simulink model "ML_UAV_3D_2"  (R2018a)
settings: Solver=ode4  StartTime=0.0  StopTime=130  FixedStep=Ts  MaxStep=2*T  MinStep=T  RelTol=1e-4
values from neighbouring files (symbols this model uses):
  Ac = 0.0331    [init_ML_UAV_3D_2.m]
  Am1_LPF = sysd.denominator{1}    [init_ML_UAV_3D_2.m]
  Am2_LPF = sysd.denominator{1}    [init_ML_UAV_3D_2.m]
  Am_coup_LPF = sysd.denominator{1}    [init_ML_UAV_3D_2.m]
  Amp_sf = 3    [init_ML_UAV_3D_2.m]
  Amp_sf_rp = 0.05*uav.m*g    [init_ML_UAV_3D_2.m]
  Bm1_LPF = sysd.numerator{1}    [init_ML_UAV_3D_2.m]
  Bm2_LPF = sysd.numerator{1}    [init_ML_UAV_3D_2.m]
  Bm_coup_LPF = sysd.numerator{1}    [init_ML_UAV_3D_2.m]
  C_S = [5;5;9]*10^-3    [init_ML_UAV_3D_2.m]
  Cd_u = 0.2    [init_ML_UAV_3D_2.m]
  dc_M_p = 6.7    [init_ML_UAV_3D_2.m]
  eps_V = 0.5    [init_ML_UAV_3D_2.m]
  g = 9.81    [init_ML_UAV_3D_2.m]
  gamma_d_p = (2*0.3/0.03*2*0.2*12/4)/10    (= 2.4)    [init_ML_UAV_3D_2.m]
  k3 = 24    [init_ML_UAV_3D_2.m]
  k4 = 0.8    [init_ML_UAV_3D_2.m]
  min_sf = 5    [init_ML_UAV_3D_2.m]
  min_sf_rp = 0.35*uav.m*g    [init_ML_UAV_3D_2.m]
  OMEGA_FILTER_OUTER = 40    [estimation.m]
  T_init = 10    [init_ML_UAV_3D_2.m]
  Tc = 1/500    (= 0.002)    [estimation.m]
  Tg = 1/ 20    (= 0.05)    [estimation.m]
  Tn = 1/500    (= 0.002)    [estimation.m]
  Ts = 1/500    (= 0.002)    [estimation.m]    (also in init_ML_UAV_3D_2.m)
  Tsc = 1/100    (= 0.01)    [estimation.m]
  Tz = 1/500    (= 0.002)    [estimation.m]
  X_GPS_offset = [0.01 0.005]    [estimation.m]
undefined symbols (not defined in the file or in its folder): Am_HPF, Am_LPF, Am_LPF2, an1, an1_v, an2, an3, Bm_HPF, Bm_LPF, Bm_LPF2, bn1, bn1_v, bn2, bn3, buoy, cable, controller, current, D_b, DiscIntNeverNeededParam, F, filters, J_u, K, kd_t, kp_t, L, Light, magnitude, MIL, Phi0, Psi0, R_b, T, Theta0, theta_q_ini, tolerences, torque_corr, uav, Vol_b, water, wave, X0_u
libraries: simulink x48, simulink_extras x10, UAV_Control x4, dspmtrx3 x2, aerolibwind2 x2
(part 4 of 6)

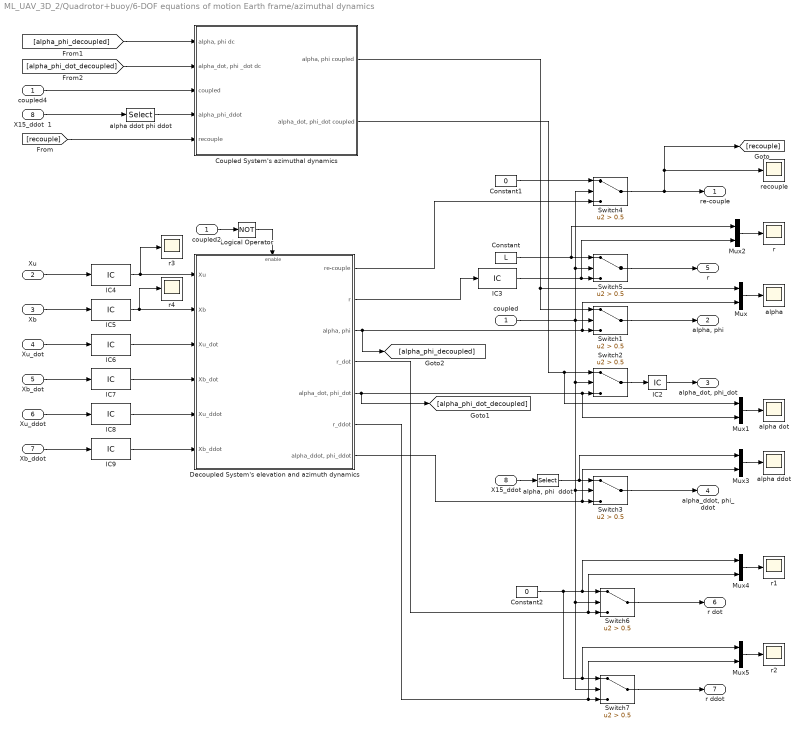
== system ML_UAV_3D_2/Quadrotor+buoy/6-DOF equations of motion Earth frame/azimuthal dynamics ==
  coupled : Inport
  Xu : Inport  Port=2
  Xb : Inport  Port=3
  "Xu_dot " : Inport  Port=4
  Xb_dot : Inport  Port=5
  Xu_ddot : Inport  Port=6
  "Xb_ddot   " : Inport  Port=7
  "X15_ddot  " : Inport  Port=8
  "    alpha ddot" : Scope
  "  alpha" : Scope
  "  alpha dot" : Scope
    r{,1..4} (5 alike) : Scope
  "  recouple   " : Scope
  Constant : Constant  Value=L
  Constant1 : Constant  Value=0
  Constant2 : Constant  Value=0
  Coupled System's azimuthal dynamics : Subsystem
  Decoupled System's elevation and azimuth dynamics : Subsystem  TreatAsAtomicUnit=on
  IC2 : InitialCondition  Value=0
  IC3 : InitialCondition  Value=r_0
  IC4 : InitialCondition  Value=pos_u_ini
  IC5 : InitialCondition  Value=pos_b_ini
  IC6 : InitialCondition  Value=v_u_ini
  IC7 : InitialCondition  Value=v_b_ini
  IC8 : InitialCondition  Value=[0; 0; 0]
  IC9 : InitialCondition  Value=[0; 0; 0]
  Logical Operator : Logic  Operator=NOT  AllPortsSameDT=off  OutDataTypeStr=boolean
  Mux{,1..5} (6 alike) : Mux  Inputs=2
  Switch{1..7} (7 alike) : Switch  Criteria=u2 > Threshold  Threshold=0.5
  X15_ddot  1 : InportShadow  Port=8
  alpha ddot phi ddot : Selector  InputPortWidth=5  IndexOptions=Index vector (dialog)  Indices=[4 5]  OutputSizes=1
  "alpha, phi  ddot" : Selector  InputPortWidth=5  IndexOptions=Index vector (dialog)  Indices=[4 5]  OutputSizes=1
  coupled2 : InportShadow
  coupled4 : InportShadow
  re-couple : Outport
  "alpha, phi" : Outport  Port=2
  "alpha_dot, phi_dot " : Outport  Port=3
  "alpha_ddot, phi_ddot" : Outport  Port=4
  "r " : Outport  Port=5
  r dot : Outport  Port=6
  r ddot : Outport  Port=7
  wires:
  coupled/1 -> Switch7/2, Switch6/2, Switch3/2, Switch2/2, Switch4/2, Switch5/2, Switch1/2
  "X15_ddot  "/1 -> "alpha, phi  ddot"/1
  Switch3/1 -> "alpha_ddot, phi_ddot"/1
  Coupled System's azimuthal dynamics/2("alpha_dot, phi_dot coupled") -> Switch2/1, Mux1/1
  Switch2/1 -> IC2/1
  Xb/1 -> IC5/1
  Xu/1 -> IC4/1
  alpha ddot phi ddot/1 -> Coupled System's azimuthal dynamics/4(alpha_phi_ddot)
  [alpha_phi_dot_decoupled] -> Coupled System's azimuthal dynamics/2("alpha_dot, phi _dot dc")
  coupled4/1 -> Coupled System's azimuthal dynamics/3(coupled)
  [alpha_phi_decoupled] -> Coupled System's azimuthal dynamics/1("alpha, phi dc")
  X15_ddot  1/1 -> alpha ddot phi ddot/1
  "Xu_dot "/1 -> IC6/1
  Xb_dot/1 -> IC7/1
  "Xb_ddot   "/1 -> IC9/1
  Xu_ddot/1 -> IC8/1
  coupled2/1 -> Logical Operator/1
  Switch5/1 -> "r "/1
  Constant/1 -> Switch5/1, Mux2/1
  Decoupled System's elevation and azimuth dynamics/2(r) -> IC3/1
  [recouple] -> Coupled System's azimuthal dynamics/5(recouple)
  Coupled System's azimuthal dynamics/1("alpha, phi coupled") -> Mux/1, Switch1/1
  Decoupled System's elevation and azimuth dynamics/7("alpha_ddot, phi_ddot") -> Mux3/2, Switch3/3
  Logical Operator/1 -> Decoupled System's elevation and azimuth dynamics/Enable
  Mux/1 -> "  alpha"/1
  Mux1/1 -> "  alpha dot"/1
  Decoupled System's elevation and azimuth dynamics/5("alpha_dot, phi_dot") -> Mux1/2, Switch2/3, [alpha_phi_dot_decoupled]
  Mux2/1 -> "  r"/1
  Decoupled System's elevation and azimuth dynamics/1(re-couple) -> Switch4/3
  Mux3/1 -> "    alpha ddot"/1
  "alpha, phi  ddot"/1 -> Mux3/1, Switch3/1
  Switch4/1 -> [recouple], "  recouple   "/1, re-couple/1
  Constant1/1 -> Switch4/1
  Switch1/1 -> "alpha, phi"/1
  IC2/1 -> "alpha_dot, phi_dot "/1
  Mux4/1 -> "  r1"/1
  Switch6/1 -> r dot/1
  Decoupled System's elevation and azimuth dynamics/4(r_dot) -> Mux4/2, Switch6/3
  Decoupled System's elevation and azimuth dynamics/6(r_ddot) -> Switch7/3, Mux5/2
  Constant2/1 -> Switch7/1, Mux5/1, Mux4/1, Switch6/1
  Switch7/1 -> r ddot/1
  Mux5/1 -> "  r2"/1
  IC3/1 -> Mux2/2, Switch5/3
  IC4/1 -> "  r3"/1, Decoupled System's elevation and azimuth dynamics/1(Xu)
  IC6/1 -> Decoupled System's elevation and azimuth dynamics/3(Xu_dot)
  IC7/1 -> Decoupled System's elevation and azimuth dynamics/4(Xb_dot)
  IC8/1 -> Decoupled System's elevation and azimuth dynamics/5(Xu_ddot)
  IC9/1 -> Decoupled System's elevation and azimuth dynamics/6(Xb_ddot)
  Decoupled System's elevation and azimuth dynamics/3("alpha, phi") -> Switch1/3, Mux/2, [alpha_phi_decoupled]
  IC5/1 -> "  r4"/1, Decoupled System's elevation and azimuth dynamics/2(Xb)

== system ML_UAV_3D_2/Quadrotor+buoy/6-DOF equations of motion Earth frame/buoyancy ==
  z_b : Inport
  zeta : Inport  Port=2
  Constant : Constant  Commented=on  Value=g*rho_w*l_b*R_b
  Manual Switch : ManualSwitch  CurrentSetting=0
  Product : Product  Commented=on
  Scope1 : Scope  Commented=on
  Scope3 : Scope  Commented=on
  V_im cuboid : Subsystem
  f(z_b,zeta) cylinder : Subsystem  Commented=on
  two connected cylindrical buoys : Gain  Commented=on  Gain=2
  two connected cylindrical buoys1 : Gain  Commented=on  Gain=l_b*R_b
  two connected cylindrical buoys2 : Gain  Commented=on  Gain=2
  V_im : Outport
  wires:
  z_b/1 -> V_im cuboid/2(zb), f(z_b,zeta) cylinder/2(zb)
  zeta/1 -> V_im cuboid/1(zeta), f(z_b,zeta) cylinder/1(zeta)
  Product/1 -> two connected cylindrical buoys/1
  Constant/1 -> Scope1/1, Product/2
  f(z_b,zeta) cylinder/1(Out1) -> two connected cylindrical buoys1/1, Product/1, Scope3/1
  Manual Switch/1 -> V_im/1
  V_im cuboid/1(Vol_im) -> Manual Switch/2
  two connected cylindrical buoys1/1 -> two connected cylindrical buoys2/1
  two connected cylindrical buoys2/1 -> Manual Switch/1

== system ML_UAV_3D_2/Quadrotor+buoy/6-DOF equations of motion Earth frame/elevation and azimuth angles to Direction Cosine Matrix Spherical to Cartesian ==
  "alpha, phi" : Inport
  -s_alpha*c_phi : Fcn  Expr=-u(1)*u(4)
  -s_alpha*s_phi : Fcn  Expr=-u(1)*u(2)
  -s_phi : Fcn  Expr=-u(2)
  Ground : Ground
  Mux : Mux  Inputs=2
  Subsystem : Subsystem
  c_alpha : Fcn  Expr=u(3)
  c_alpha*c_phi : Fcn  Expr=u(3)*u(4)
  c_alpha*s_phi : Fcn  Expr=u(3)*u(2)
  c_phi : Fcn  Expr=u(4)
  s_alpha : Fcn  Expr=u(1)
  sincos : Trigonometry  Operator=sincos
  DCM : Outport  PortDimensions=[3,3]
  wires:
  -s_alpha*c_phi/1 -> Subsystem/2(In2)
  -s_phi/1 -> Subsystem/3(In3)
  Subsystem/1(Out1) -> DCM/1
  c_alpha/1 -> Subsystem/8(In8)
  sincos/2 -> Mux/2
  s_alpha/1 -> Subsystem/7(In7)
  c_alpha*s_phi/1 -> Subsystem/4(In4)
  Ground/1 -> Subsystem/9(In9)
  Mux/1 -> c_alpha*s_phi/1, s_alpha/1, c_alpha/1, c_phi/1, -s_alpha*s_phi/1, -s_phi/1, -s_alpha*c_phi/1, c_alpha*c_phi/1
  -s_alpha*s_phi/1 -> Subsystem/5(In5)
  c_alpha*c_phi/1 -> Subsystem/1(In1)
  c_phi/1 -> Subsystem/6(In6)
  sincos/1 -> Mux/1
  "alpha, phi"/1 -> sincos/1

== system ML_UAV_3D_2/Quadrotor+buoy/6-DOF equations of motion Earth frame/u123 ==
  u1 : Inport
  euler_u : Inport  Port=2
  V_im : Inport  Port=3
  a_p : Inport  Port=4
  coupled : Inport  Port=5
  -s_alpha*c_phi : Fcn  Expr=-u(1)*u(4)
  -s_alpha*s_phi : Fcn  Expr=-u(1)*u(2)
  Add : Sum
  Add1 : Sum  Inputs=3
  Constant1 : Constant  Value=rho_w*g
  Constant2 : Constant  Commented=on  Value=Vol_b/2
  F_B : Product
  Gain : Gain  Gain=L
  Gain1 : Gain  Gain=L
  Mux : Mux  Inputs=2
  Mux1 : Mux  Inputs=2
  Mux2 : Mux  Inputs=3
  Product1 : Product  Inputs=3  SaturateOnIntegerOverflow=on  InputSameDT=on  OutDataTypeStr=Inherit: Same as first input
  Product{2..10} (9 alike) : Product  Inputs=**  SaturateOnIntegerOverflow=on  InputSameDT=on  OutDataTypeStr=Inherit: Same as first input
  Product11 : Product  Inputs=3  SaturateOnIntegerOverflow=on  InputSameDT=on  OutDataTypeStr=Inherit: Same as first input
  Scope{1..4,9} (5 alike) : Scope
  Signal Specification2 : SignalSpecification  Dimensions=5
  Sum1 : Sum  Inputs=|++  SaturateOnIntegerOverflow=on
  Vector Concatenate3 : Concatenate  NumInputs=5
  c_alpha : Fcn  Expr=u(3)
  c_phi : Fcn  Expr=u(4)
  c_phi c_theta : Fcn  Expr=u(4)*u(5)
  coupled1 : InportShadow  Port=5
  s_phi : Fcn  Expr=-u(2)
  s_theta c_psi + s_phi c_theta s_psi : Fcn  Expr=u(1)*u(5)*u(3) + u(2)*u(6)
  s_theta s_psi - s_phi c_theta c_psi : Fcn  Expr=-u(1)*u(5)*u(6) + u(2)*u(3)
  sincos : Trigonometry  Operator=sincos
  sincos1 : Trigonometry  Operator=sincos
  "u1 " : InportShadow
  u15 : Outport
  R_u_3 : Outport  Port=2
  wires:
  Product7/1 -> Sum1/1
  Product2/1 -> Product7/1, Product3/1, Product6/1
  Product1/1 -> Vector Concatenate3/4
  Vector Concatenate3/1 -> Scope9/1, Signal Specification2/1
  Product6/1 -> Vector Concatenate3/1
  Sum1/1 -> Vector Concatenate3/3
  F_B/1 -> Sum1/2
  V_im/1 -> F_B/1
  Gain/1 -> Product1/2
  Constant1/1 -> F_B/2
  Signal Specification2/1 -> u15/1
  coupled/1 -> Product2/1
  u1/1 -> Product2/2
  "u1 "/1 -> Product11/3, Product1/3
  Mux/1 -> c_phi c_theta/1, s_theta s_psi - s_phi c_theta c_psi/1, s_theta c_psi + s_phi c_theta s_psi/1
  sincos/1 -> Mux/1
  sincos/2 -> Mux/2
  euler_u/1 -> sincos/1
  s_theta c_psi + s_phi c_theta s_psi/1 -> Product9/1, Scope3/1, Product4/1, Mux2/1, Product6/2  "R_31"
  s_theta s_psi - s_phi c_theta c_psi/1 -> Scope4/1, Product10/1, Product5/1, Mux2/2, Product3/2  "R_32"
  Product3/1 -> Vector Concatenate3/2
  c_phi c_theta/1 -> Product8/1, Mux2/3, Product7/2  "R_33"
  a_p/1 -> sincos1/1
  sincos1/1 -> Mux1/1
  sincos1/2 -> Mux1/2
  Mux1/1 -> c_phi/1, s_phi/1, c_alpha/1, -s_alpha*s_phi/1, -s_alpha*c_phi/1
  -s_alpha*c_phi/1 -> Product4/2
  Product4/1 -> Add1/1
  Product5/1 -> Add1/2
  -s_alpha*s_phi/1 -> Product5/2
  Product8/1 -> Add1/3
  c_alpha/1 -> Product8/2
  Product9/1 -> Scope2/1, Add/1
  Product10/1 -> Scope1/1, Add/2
  s_phi/1 -> Product9/2
  c_phi/1 -> Product10/2
  Add1/1 -> Gain/1
  coupled1/1 -> Product11/1, Product1/1
  Gain1/1 -> Product11/2
  Product11/1 -> Vector Concatenate3/5
  Add/1 -> Gain1/1
  Mux2/1 -> R_u_3/1

== system ML_UAV_3D_2/Sensors and Filters/Coupling detection by r/Coupling state ==
  r_est : Inport
  re_couple : Inport  Port=2
  Data Type Conversion : DataTypeConversion  OutDataTypeStr=double
  Delay10 : Delay  DelayLength=1  InitialCondition=0
  IC3 : InitialCondition  Value=0
  IC5 : InitialCondition  Value=0
  MATLAB Function : MATLAB Function  TreatAsAtomicUnit=on
  "T, r,xu,xb1" : Scope
  break algebraic loop : Delay  DelayLength=1  InitialCondition=1
  cable length with safety margine1 : simulink/Logic and Bit Operations/Compare To Constant  relop=>=  const=cable.L_0-0.05  OutDataTypeStr=boolean
  "is coupled " : Scope
  is coupled -1 : Scope
  pos tension : Scope
  positive tension : Scope
  "re_couple " : Scope
  state detector : Scope
  is coupled : Outport
  wires:
  Delay10/1 -> is coupled -1/1, MATLAB Function/3(coupled)
  IC5/1 -> is coupled/1, Delay10/1
  MATLAB Function/1(is_coupled) -> IC5/1, "is coupled "/1
  break algebraic loop/1 -> pos tension/1, MATLAB Function/1(pos_T)
  re_couple/1 -> MATLAB Function/2(re_couple), "re_couple "/1
  MATLAB Function/2(c) -> state detector/1
  Data Type Conversion/1 -> positive tension/1, break algebraic loop/1
  IC3/1 -> Data Type Conversion/1
  cable length with safety margine1/1 -> IC3/1
  r_est/1 -> "T, r,xu,xb1"/1, cable length with safety margine1/1

== system ML_UAV_3D_2/Sensors and Filters/Data processing/Estimate Attitude ==
  Acc : Inport
  q : Inport  Port=2
  Euler : Inport  Port=3
  Calculate Roll and Pitch (From Acceleration Data) : Subsystem
  Constant : Constant  Value=Ts
  Demux : Demux  Outputs=2
  Ground : Ground
  High Pass Filter1 : DiscreteTransferFcn  Numerator=Bm_HPF  Denominator=Am_HPF
  Kalman Filter - Pitch : MATLAB Function  TreatAsAtomicUnit=on
  Manual Switch1 : ManualSwitch  CurrentSetting=0
  Mux : Mux  Inputs=3
  Mux2 : Mux  Inputs=2
  Mux5 : Mux  Inputs=2
  Notch Filter1 : Subsystem
  Scope1 : Scope
  Signal Specification : SignalSpecification  Dimensions=1
  theta : Scope
  q_g : Outport
  q_f : Outport  Port=2
  " pitch" : Outport  Port=3
  wires:
  q/1 -> High Pass Filter1/1, Mux2/2
  Notch Filter1/2(q) -> Kalman Filter - Pitch/2(gyro_rate), q_f/1
  Calculate Roll and Pitch (From Acceleration Data)/1(pitch_acc (rad)) -> Kalman Filter - Pitch/1(acc_angle)
  Signal Specification/1 -> " pitch"/1  "Kalman"
  Euler/1 -> Mux5/1, Kalman Filter - Pitch/3(opti_angle)  "pitch"
  Constant/1 -> Kalman Filter - Pitch/4(dt)
  Acc/1 -> Demux/1
  Notch Filter1/1(y) -> Manual Switch1/2
  High Pass Filter1/1 -> Manual Switch1/1, Notch Filter1/1(u), Mux2/1
  Mux2/1 -> Scope1/1
  Kalman Filter - Pitch/1(angle) -> Mux5/2, Signal Specification/1
  Mux/1 -> Calculate Roll and Pitch (From Acceleration Data)/1(accel (m/s^2) [3])
  Demux/1 -> Mux/1
  Demux/2 -> Mux/3
  Ground/1 -> Mux/2
  Manual Switch1/1 -> q_g/1
  Mux5/1 -> theta/1

== system ML_UAV_3D_2/Sensors and Filters/Data processing/Estimate Position ==
  OptiTrack : Inport
  "pitch, Kalman" : Inport  Port=2
  Sonar : Inport  Port=3
  2nd Order Filter : Subsystem
  2nd Order Filter2 : Subsystem
  2nd Order Filter4 : Subsystem
  2nd Order Filter5 : Subsystem
  Constant4 : Constant  Value=Tc
  Demux2 : Demux
  Extrapolation - x : MATLAB Function  TreatAsAtomicUnit=on
  Extrapolation - z : MATLAB Function  TreatAsAtomicUnit=on
  Height est : Scope
  Height est1 : Scope
  Kalman Filter - Height : MATLAB Function  TreatAsAtomicUnit=on
  Manual Switch : ManualSwitch  CurrentSetting=0
  Mux : Mux  Inputs=2
  Mux1 : Mux  Inputs=2
  Mux2 : Mux  Inputs=3
  Mux3 : Mux  Inputs=3
  Mux4 : Mux  Inputs=3
  Notch Filter2 : Subsystem
  Position : Selector  InputPortWidth=5  IndexOptions=Index vector (dialog)  Indices=[1 2 4 5]  OutputSizes=1
  Signal Conditioning - Sonar : Subsystem
  Signal Specification : SignalSpecification  Dimensions=2
  Signal Specification1 : SignalSpecification  Dimensions=2
  Step Size : Constant  Value=Tc
  Step Size1 : Constant  Value=X0_u(1)
  Step Size2 : Constant  Value=X0_u(2)
  Step Size3 : Constant  Value=X0_u(2)
  Terminator1 : Terminator
  Terminator2 : Terminator
  Thrust1 : Scope
  Thrust11 : Scope
  V_est : Scope  Commented=on
  X_est : Scope  Commented=on
  Xe : Outport
  Ve : Outport  Port=2
  wires:
  Demux2/1 -> Mux3/1, Extrapolation - x/1(xin)
  2nd Order Filter5/2(yd) -> [height_rate_Kalman]
  Demux2/3 -> Extrapolation - x/4(new), Extrapolation - z/4(new)  "New Data"
  Constant4/1 -> Kalman Filter - Height/3(dt)
  Extrapolation - x/1(xout) -> Mux3/2, 2nd Order Filter/1(u)
  2nd Order Filter/1(y) -> Mux3/3, Mux/1
  2nd Order Filter4/2(yd) -> Kalman Filter - Height/2(sonar_d)
  2nd Order Filter2/1(y) -> Mux4/3, Kalman Filter - Height/1(optitrack), Mux2/2
  Sonar/1 -> Signal Conditioning - Sonar/1(sonar (m))
  2nd Order Filter4/1(y) -> Terminator1/1
  Signal Conditioning - Sonar/1(calib sonar (m)) -> Mux2/1, 2nd Order Filter4/1(u)
  Step Size/1 -> Extrapolation - z/3(dt), Extrapolation - x/3(dt)
  Position/1 -> Demux2/1
  Demux2/2 -> Mux4/1, Extrapolation - z/1(xin)
  2nd Order Filter5/1(y) -> Terminator2/1
  Mux/1 -> Signal Specification/1  "Xe IMU or GPS"
  [height_rate_Kalman] -> Mux1/2
  Demux2/4 -> Extrapolation - x/5(isTracking), Extrapolation - z/5(isTracking)  "Is Tracking"
  Mux2/1 -> Height est/1
  Mux1/1 -> Signal Specification1/1  "Ve IMU or GPS"
  OptiTrack/1 -> Thrust1/1, Position/1
  Mux3/1 -> Thrust11/1
  2nd Order Filter2/2(yd) -> Extrapolation - z/2(xdotin)
  Notch Filter2/1(y) -> Manual Switch/2
  2nd Order Filter/2(yd) -> Notch Filter2/1(u), Manual Switch/1, Extrapolation - x/2(xdotin)
  Manual Switch/1 -> Mux1/1
  Signal Specification/1 -> Xe/1, X_est/1
  Signal Specification1/1 -> Ve/1, V_est/1
  Kalman Filter - Height/1(height) -> [height_Kalman], Mux2/3, 2nd Order Filter5/1(u)
  [height_Kalman] -> Mux/2
  "pitch, Kalman"/1 -> Signal Conditioning - Sonar/2(pitch (rad))
  Mux4/1 -> Height est1/1
  Extrapolation - z/1(xout) -> Mux4/2, 2nd Order Filter2/1(u)
  Step Size1/1 -> Extrapolation - x/6(x0)
  Step Size2/1 -> Extrapolation - z/6(x0)
  Step Size3/1 -> Kalman Filter - Height/4(x0)

== system ML_UAV_3D_2/Sensors and Filters/Sensors/ Sonar (10Hz) (true elevation instead real sonar signal) ==
  note: "Smooth" out the Sonar data
  note: Resample the 10Hz Sonar Data
  sonar (m) : Inport
  FOH1 : Subsystem  mask{Ts=0.1}
      mask prompts: Ts "Sample Time"
  IC : InitialCondition  Value=X0_u(2)
  Rate Transition : RateTransition  InitialCondition=X0_u(2)
  Sampler : Subsystem  mask{Ts=0.1}
      mask prompts: Ts "Sample Time"
  calib sonar (m) : Outport
  wires:
  Sampler/1(Out1) -> Rate Transition/1
  Rate Transition/1 -> FOH1/1(Input)
  sonar (m)/1 -> Sampler/1(In1)
  FOH1/1(Output) -> IC/1
  IC/1 -> calib sonar (m)/1

== system ML_UAV_3D_2/Sensors and Filters/Sensors/Accelerometer (500Hz) ==
  Ab : Inport
  "Ab " : Scope  Commented=on
  Demux1 : Demux  Outputs=2
  From File : FromFile  FileName=acc_x_noise.mat  SampleTime=Tz
  From File2 : FromFile  FileName=acc_z_noise.mat  SampleTime=Tz
  IC : InitialCondition  Value=[0 0]
  Manual Switch{,2,4,6} (4 alike) : ManualSwitch
  Mux1 : Mux  Inputs=2
  Mux2 : Mux  Inputs=2
  Product : Product  SaturateOnIntegerOverflow=on  RndMeth=Zero  InputSameDT=on  OutDataTypeStr=Inherit: Same as first input
  Product2 : Product  SaturateOnIntegerOverflow=on  RndMeth=Zero  InputSameDT=on  OutDataTypeStr=Inherit: Same as first input
  Slider Gain : simulink/Math Operations/Slider Gain  gain=1  low=0  high=2
  Slider Gain2 : simulink/Math Operations/Slider Gain  gain=1  low=0  high=2
  Sum2 : Sum  Inputs=+++  SaturateOnIntegerOverflow=on  InputSameDT=on  OutDataTypeStr=Inherit: Same as first input
  Sum5 : Sum  Inputs=+++  SaturateOnIntegerOverflow=on  InputSameDT=on  OutDataTypeStr=Inherit: Same as first input
  acc_noisy : Scope  Commented=on
  bias : Constant  Value=0.05  VectorParams1D=off
  bias10 : Constant  Value=1.02  VectorParams1D=off
  bias11 : Constant  VectorParams1D=off
  bias3 : Constant  Value=1.02  VectorParams1D=off
  bias4 : Constant  VectorParams1D=off
  bias6 : Constant  Value=0  VectorParams1D=off
  bias7 : Constant  Value=0.05  VectorParams1D=off
  bias8 : Constant  Value=0  VectorParams1D=off
  Acc : Outport
  wires:
  bias11/1 -> Manual Switch6/2
  bias10/1 -> Manual Switch6/1
  bias4/1 -> Manual Switch4/2
  bias3/1 -> Manual Switch4/1
  Manual Switch2/1 -> Sum2/2
  bias8/1 -> Manual Switch2/2
  bias7/1 -> Manual Switch2/1
  bias6/1 -> Manual Switch/2
  bias/1 -> Manual Switch/1
  Manual Switch/1 -> Sum5/2
  Manual Switch6/1 -> Product2/1
  Manual Switch4/1 -> Product/1
  Product2/1 -> Mux1/2
  Sum2/1 -> Product2/2
  Product/1 -> Mux1/1
  Sum5/1 -> Product/2
  From File2/1 -> Slider Gain2/1
  Demux1/1 -> Sum5/3
  Demux1/2 -> Sum2/3
  From File/1 -> Slider Gain/1
  Mux2/1 -> acc_noisy/1
  Mux1/1 -> IC/1
  Ab/1 -> Demux1/1, Mux2/2, "Ab "/1
  Slider Gain/1 -> Sum5/1
  Slider Gain2/1 -> Sum2/1
  IC/1 -> Mux2/1, Acc/1

== system ML_UAV_3D_2/Sensors and Filters/Sensors/GPS (10Hz)  ==
  note: 0.2
  Xe : Inport
  Euler : Inport  Port=2
  DCM_b2e : Inport  Port=3
  Constant : Constant  Value=X_GPS_offset
  Constant1 : Constant
  Demux : Demux  Outputs=2
  IC : InitialCondition  Value=[X0_u Theta0]
  Is Tracking : simulink/Sources/Repeating Sequence Stair  Commented=on  OutValues=[1 1 1 1 1 1 1 1 1 1 1 1 1 1 1 1 1 1 1 1]  tsamp=To  OutMin=[]  OutMax=[]  OutDataTypeStr=double  OutputDataTypeScalingMode=double  OutDataType=fixdt(0,8)  ConRadixGroup=Best Precision: Vector-wise  OutScaling=2^-12
  Logical Operator : Logic  AllPortsSameDT=off  OutDataTypeStr=boolean
  Mux : Mux  Inputs=3
  Mux1 : Mux  Inputs=3
  New Data : simulink/Sources/Repeating Sequence Stair  Commented=on  OutValues=[1 1 1 0 0 1 0 1 1 1 1 0 1 1 0 1 1 1 1 1 0 0 0 1 1 0 1 1 1 0]  tsamp=To  OutMin=[]  OutMax=[]  OutDataTypeStr=double  OutputDataTypeScalingMode=double  OutDataType=fixdt(0,8)  ConRadixGroup=Best Precision: Vector-wise  OutScaling=2^-12
  Product : Product  Multiplication=Matrix(*)
  Random Number : RandomNumber  Variance=5/10000  SampleTime=Tg
  Random Number2 : RandomNumber  Variance=5/10000  SampleTime=Tg
  Random Number4 : RandomNumber  Variance=1/100000  SampleTime=Tg
  Rate Transition : RateTransition
  Rate Transition2 : RateTransition
  Rate Transition4 : RateTransition
  Scope : Scope  Commented=on
  Slider Gain : simulink/Math Operations/Slider Gain  gain=0.5  low=0  high=2
  Slider Gain2 : simulink/Math Operations/Slider Gain  gain=0.5  low=0  high=2
  Slider Gain4 : simulink/Math Operations/Slider Gain  gain=1  low=0  high=2
  Sum : Sum  Inputs=++|
  Sum2 : Sum  Inputs=++|
  Sum4 : Sum  Inputs=++|
  Sum6 : Sum  Inputs=|++
  Switch : Switch  Criteria=u2 > Threshold  Threshold=0.5
  Variable Integer Delay1 : Delay  DelayLength=1
  Variable Integer Delay3 : Delay  DelayLength=1  InitialCondition=[X0_u Theta0]
  optiTrack : Scope  Commented=on
  optiTrack1 : Scope  Commented=on
  optiTrack2 : Scope
  optiTrack3 : Scope
  optiTrack4 : Scope
  GPS : Outport
  wires:
  Mux/1 -> Variable Integer Delay3/1
  Constant1/1 -> Mux1/2, Logical Operator/1, Mux1/3, Logical Operator/2
  Logical Operator/1 -> optiTrack1/1, Switch/2
  Variable Integer Delay1/1 -> Switch/3
  Slider Gain/1 -> Sum2/1
  Random Number2/1 -> Rate Transition2/1
  Demux/1 -> Sum/2
  Demux/2 -> Sum2/2
  Sum2/1 -> Mux/2
  Sum/1 -> Mux/1
  Random Number/1 -> Rate Transition/1
  Slider Gain2/1 -> optiTrack2/1, Sum/1
  Mux1/1 -> GPS/1
  Random Number4/1 -> Rate Transition4/1
  Euler/1 -> Sum4/2
  Sum4/1 -> Mux/3
  Variable Integer Delay3/1 -> Switch/1, optiTrack3/1
  Rate Transition/1 -> Slider Gain2/1
  Rate Transition2/1 -> Scope/1, Slider Gain/1
  Rate Transition4/1 -> Slider Gain4/1
  Switch/1 -> Variable Integer Delay1/1, IC/1  "x,z,theta"
  Sum6/1 -> Demux/1
  DCM_b2e/1 -> Product/1
  Constant/1 -> Product/2
  Product/1 -> Sum6/2
  Xe/1 -> Sum6/1
  IC/1 -> optiTrack/1, Mux1/1
  Slider Gain4/1 -> Sum4/1, optiTrack4/1

== system ML_UAV_3D_2/Sensors and Filters/Sensors/Gyro (500Hz) ==
  q : Inport
  Degrees to Radians2 : simulink_extras/Transformations/Degrees to Radians
  From File1 : FromFile  FileName=gyro_q_noise.mat  SampleTime=Tz
  Manual Switch1 : ManualSwitch
  Manual Switch5 : ManualSwitch  CurrentSetting=0
  Product1 : Product  SaturateOnIntegerOverflow=on  RndMeth=Zero  InputSameDT=on  OutDataTypeStr=Inherit: Same as first input
  Slider Gain1 : simulink/Math Operations/Slider Gain  gain=1  low=0  high=2
  Sum2 : Sum  Inputs=+++  SaturateOnIntegerOverflow=on  InputSameDT=on  OutDataTypeStr=Inherit: Same as first input
  Variable Integer Delay3 : Delay  DelayLength=0
  bias1 : Constant  Value=-1  VectorParams1D=off
  bias2 : Constant  Value=0  VectorParams1D=off
  bias5 : Constant  Value=0.9  VectorParams1D=off
  bias9 : Constant  VectorParams1D=off
  " q" : Outport
  wires:
  bias9/1 -> Manual Switch5/2
  bias5/1 -> Manual Switch5/1
  Manual Switch1/1 -> Degrees to Radians2/1
  bias2/1 -> Manual Switch1/2
  bias1/1 -> Manual Switch1/1
  Degrees to Radians2/1 -> Sum2/2
  Manual Switch5/1 -> Product1/1
  Sum2/1 -> Product1/2
  From File1/1 -> Slider Gain1/1
  Product1/1 -> Variable Integer Delay3/1
  Variable Integer Delay3/1 -> " q"/1
  Slider Gain1/1 -> Sum2/1
  q/1 -> Sum2/3

== system ML_UAV_3D_2/Sensors and Filters/Sensors/rotation matrix R ==
  angle (rad) : Inport
  Gain : Gain  Gain=-1
  Signal Specification1 : SignalSpecification  Dimensions=2
  Signal Specification2 : SignalSpecification  Dimensions=2
  Trigonometric Function1 : Trigonometry  Operator=sincos
  Vector Concatenate1 : Concatenate  Mode=Multidimensional array  ConcatenateDimension=2
  Vector Concatenate2 : Concatenate
  Vector Concatenate3 : Concatenate
  R : Outport
  wires:
  Signal Specification2/1 -> Vector Concatenate1/2
  Signal Specification1/1 -> Vector Concatenate1/1
  Vector Concatenate1/1 -> R/1
  Vector Concatenate2/1 -> Signal Specification1/1
  Vector Concatenate3/1 -> Signal Specification2/1
  angle (rad)/1 -> Trigonometric Function1/1
  Trigonometric Function1/2 -> Vector Concatenate3/2, Vector Concatenate2/1
  Trigonometric Function1/1 -> Vector Concatenate2/2, Gain/1
  Gain/1 -> Vector Concatenate3/1

== system ML_UAV_3D_2/UAV controller/Attitutde Control/UAV inner loop control ==
  theta_d : Inport
  theta_q : Inport  Port=2
  omega_q : Inport  Port=3
  Constant : Constant  Value=J_u
  Discrete Transfer Fcn : DiscreteTransferFcn  Numerator=Bm1_LPF  Denominator=Am1_LPF
  Discrete Transfer Fcn1 : DiscreteTransferFcn  Numerator=Bm2_LPF  Denominator=Am2_LPF
  Discrete Derivative3 : simulink/Discrete/Discrete Derivative  gainval=1.0  ICPrevScaledInput=Theta0/T  OutMin=[]  OutMax=[]  OutDataType=fixdt(1, 16)  OutScaling=2^-10  DoSatur=off
  Discrete Derivative4 : simulink/Discrete/Discrete Derivative  gainval=1.0  ICPrevScaledInput=0.0  OutMin=[]  OutMax=[]  OutDataType=fixdt(1, 16)  OutScaling=2^-10  DoSatur=off
  Discrete Derivative6 : simulink/Discrete/Discrete Derivative  gainval=1.0  ICPrevScaledInput=Theta0/T  OutMin=[]  OutMax=[]  OutDataType=fixdt(1, 16)  OutScaling=2^-10  DoSatur=off
  Discrete-Time Integrator : DiscreteIntegrator  SampleTime=-1  LimitOutput=on  UpperSaturationLimit=dc_M_p  LowerSaturationLimit=-dc_M_p  ICPrevOutput=DiscIntNeverNeededParam  ICPrevScaledInput=DiscIntNeverNeededParam
  Gain : Gain  Gain=gamma_d_p
  IC : InitialCondition  Value=0
  IC2 : InitialCondition  Value=0
  Integrator : Integrator  Commented=on  LimitOutput=on  UpperSaturationLimit=dc_M_p  LowerSaturationLimit=-dc_M_p
  K1 : Gain  Gain=kp_t
  K2 : Gain  Gain=kd_t
  K3 : Gain  Gain=1+k3*k4
  K4 : Gain  Gain=k3+k4
  K5 : Gain
  K6 : Gain
  Mux : Mux  Inputs=2
  Mux1 : Mux  Inputs=3
  Mux2 : Mux  Inputs=2
  Product1 : Product
  Saturation : Saturate  UpperLimit=[5]  LowerLimit=[-5]
  Saturation - Limit Height Controller1 : Saturate  UpperLimit=K*L*torque_corr/4  LowerLimit=-K*L*torque_corr/4
  Saturation - Limit Height Controller2 : Saturate  UpperLimit=15  LowerLimit=-15
  Sum : Sum  Inputs=|+-
  Sum1 : Sum  Inputs=|+-
  Sum4 : Sum  Inputs=--+-
  T2 {,1..9} (10 alike) : Scope
  theta_d1 : InportShadow
  M1 (N.m) : Outport
  wires:
  Product1/1 -> Saturation - Limit Height Controller1/1
  Saturation - Limit Height Controller1/1 -> "T2 "/1, M1 (N.m)/1
  Sum1/1 -> K2/1  "ev"
  Sum4/1 -> Product1/1
  Discrete Derivative6/1 -> IC/1
  Discrete Derivative3/1 -> IC2/1
  Discrete Transfer Fcn1/1 -> Mux2/1, Saturation/1
  Sum/1 -> K1/1, Discrete-Time Integrator/1  "ex"
  K1/1 -> T2 7/1, Sum4/1
  K2/1 -> K6/1
  Discrete-Time Integrator/1 -> Gain/1
  Gain/1 -> K5/1, T2 5/1
  Constant/1 -> Product1/2
  Mux/1 -> T2 1/1
  theta_q/1 -> Mux/1, Sum/1
  omega_q/1 -> Mux1/1, Sum1/1
  Mux1/1 -> T2 2/1
  Discrete Transfer Fcn/1 -> Mux1/2, Sum1/2  "ex"
  Discrete Derivative4/1 -> Mux2/2, Discrete Transfer Fcn1/1, T2 3/1
  theta_d/1 -> Mux/2, Sum/2, Discrete Derivative6/1
  Saturation/1 -> T2 8/1, Sum4/3
  IC/1 -> Mux1/3, Discrete Transfer Fcn/1
  theta_d1/1 -> Discrete Derivative3/1
  IC2/1 -> Discrete Derivative4/1
  K5/1 -> Sum4/4
  Mux2/1 -> T2 4/1
  K6/1 -> T2 6/1, Sum4/2

== system ML_UAV_3D_2/UAV controller/u_r_p_Lyapunov radial position2/nu_x, buoy surge velocity controller ==
  note: (this is an augmentation
      | to the nominal controller
      | for better drag compensation
      | [error in tension estimation])
  note: u_x feedback, buoy surge velocity controller
  ex dot : Inport
  coupled : Inport  Port=2
  V_bar : Inport  Port=3
  integral reset : Inport  Port=4
  Enable : EnablePort
  Add1 : Sum
  Bias : Bias  Bias=0.5
  Constant1 : Constant  Value=0
  Discrete-Time Integrator1 : DiscreteIntegrator  ExternalReset=level  SampleTime=-1  LimitOutput=on  UpperSaturationLimit=10  LowerSaturationLimit=-10  ICPrevOutput=DiscIntNeverNeededParam  ICPrevScaledInput=DiscIntNeverNeededParam
  Gain11 : Gain  Gain=controller.gains.nux.ki
  Gain3 : Gain  Gain=0.5
  Gain4 : Gain  Gain=controller.gains.nux.kp
  Mux7 : Mux  Inputs=3
  Product4 : Product
  Product6 : Product
  Saturation4 : Saturate  UpperLimit=5  LowerLimit=1
  "[-22 m_u, 22 m_u]" : Saturate  UpperLimit=22.2*uav.m  LowerLimit=-22.2*uav.m
  smooth switch : Subsystem
  tuner3 : Gain
  "ur,c, PI, fb" : Scope
  "ur_c_feedback " : Scope
  ux_c : Outport
  wires:
  tuner3/1 -> "[-22 m_u, 22 m_u]"/1
  V_bar/1 -> Saturation4/1
  integral reset/1 -> smooth switch/3(switch), Discrete-Time Integrator1/2
  Add1/1 -> Mux7/3, Product4/1
  Gain3/1 -> Bias/1
  Product6/1 -> Gain11/1, Gain4/1
  Product4/1 -> tuner3/1
  Discrete-Time Integrator1/1 -> smooth switch/1(u 1)
  Bias/1 -> Product6/2
  smooth switch/1(y) -> Mux7/2, Add1/2
  ex dot/1 -> Product6/1
  "[-22 m_u, 22 m_u]"/1 -> ux_c/1, "ur_c_feedback "/1
  Saturation4/1 -> Product4/2
  Constant1/1 -> smooth switch/2(u 2)
  Gain4/1 -> Mux7/1, Add1/1
  Gain11/1 -> Discrete-Time Integrator1/1
  Mux7/1 -> "ur,c, PI, fb"/1
  coupled/1 -> Gain3/1

== system ML_UAV_3D_2/UAV controller/u_r_p_Lyapunov radial position2/output conditioning ==
  U_in : Inport
  switch : Inport  Port=2
  Demux : Demux  Outputs=3
  Mux3 : Mux  Inputs=3
  Saturation1 : Saturate  UpperLimit=1  LowerLimit=-1
  Subsystem1 : Subsystem
  smooth lower bound2 : Subsystem
  smooth switching with memory : Subsystem
  U_out : Outport
  wires:
  U_in/1 -> Demux/1
  switch/1 -> smooth switching with memory/2(switch), Subsystem1/1(switch)
  Demux/1 -> Subsystem1/2(u_r)  "u1"
  Demux/3 -> Saturation1/1  "u3"
  smooth lower bound2/1(sat(u)) -> Mux3/2
  Demux/2 -> smooth lower bound2/1(u)  "u2"
  Subsystem1/1(Out1) -> Mux3/1
  Mux3/1 -> smooth switching with memory/1(u)
  smooth switching with memory/1(y) -> U_out/1
  Saturation1/1 -> Mux3/3

== system ML_UAV_3D_2/UAV controller/u_r_p_Lyapunov radial position2/u_alpha, both controllers ==
  note: Decoupled
  note: Coupled
  note: u_alpha feedback, both controllers
  e_alpha : Inport
  e_alpha_dot : Inport  Port=2
  pulling flag : Inport  Port=3
  Add4 : Sum  Inputs=3
  Constant : Constant  Value=controller.gains.alpha.kp
  Constant1 : Constant  Value=controller.gains.alpha.ki
  Constant2 : Constant  Value=controller.gains.alpha.kd
  Constant3 : Constant  Value=controller.gains.alpha.kp
  Constant4 : Constant  Value=controller.gains.alpha.ki
  Constant5 : Constant  Value=controller.gains.alpha.kd
  Demux : Demux  Outputs=3
  Discrete-Time Integrator : DiscreteIntegrator  SampleTime=-1  LimitOutput=on  UpperSaturationLimit=2  LowerSaturationLimit=-2  ICPrevOutput=DiscIntNeverNeededParam  ICPrevScaledInput=DiscIntNeverNeededParam
  Mux : Mux  Inputs=3
  Mux1 : Mux  Inputs=3
  Product : Product
  Product1 : Product
  Product2 : Product
  Saturation1 : Saturate  UpperLimit=7  LowerLimit=-7
  Saturation3 : Saturate  UpperLimit=30*3.14/180  LowerLimit=-30*3.14/180
  pid_fb : Scope  NumInputPorts=4
  smooth switch : Subsystem
  tuner1 : Gain
  ua_c,dc : Outport
  wires:
  tuner1/1 -> ua_c,dc/1
  Saturation3/1 -> Product/2
  Saturation1/1 -> Product2/2
  Product/1 -> pid_fb/1, Add4/1  "p"
  Product2/1 -> pid_fb/3, Add4/3  "d"
  Add4/1 -> tuner1/1, pid_fb/4  "fb"
  e_alpha_dot/1 -> Saturation1/1
  Product1/1 -> Discrete-Time Integrator/1
  Discrete-Time Integrator/1 -> pid_fb/2, Add4/2  "i"
  Constant/1 -> Mux/1
  Constant1/1 -> Mux/2
  Constant2/1 -> Mux/3
  Constant4/1 -> Mux1/2
  Constant3/1 -> Mux1/1
  Constant5/1 -> Mux1/3
  pulling flag/1 -> smooth switch/3(switch)
  Mux1/1 -> smooth switch/1(u 1)
  Mux/1 -> smooth switch/2(u 2)
  smooth switch/1(y) -> Demux/1
  Demux/1 -> Product/1
  e_alpha/1 -> Saturation3/1, Product1/2
  Demux/2 -> Product1/1
  Demux/3 -> Product2/1

== system ML_UAV_3D_2/UAV controller/u_r_p_Lyapunov radial position2/u_alpha, both controllers1 ==
  note: Decoupled
  note: Coupled
  note: u_alpha feedback, both controllers
  e_phi : Inport
  e_phi_dot : Inport  Port=2
  pulling flag : Inport  Port=3
  Add4 : Sum  Inputs=3
  Constant : Constant  Value=controller.gains.phi.kp
  Constant1 : Constant  Value=controller.gains.phi.ki
  Constant2 : Constant  Value=controller.gains.phi.kd
  Constant3 : Constant  Value=controller.gains.phi.kp
  Constant4 : Constant  Value=controller.gains.phi.ki
  Constant5 : Constant  Value=controller.gains.phi.kd
  Demux : Demux  Outputs=3
  Discrete-Time Integrator : DiscreteIntegrator  SampleTime=-1  LimitOutput=on  UpperSaturationLimit=1  LowerSaturationLimit=-1  ICPrevOutput=DiscIntNeverNeededParam  ICPrevScaledInput=DiscIntNeverNeededParam
  Mux : Mux  Inputs=3
  Mux1 : Mux  Inputs=3
  Product : Product
  Product1 : Product
  Product2 : Product
  Saturation1 : Saturate  UpperLimit=7  LowerLimit=-7
  Saturation3 : Saturate  UpperLimit=7*3.14/180  LowerLimit=-7*3.14/180
  pid_fb : Scope  NumInputPorts=4
  smooth switch : Subsystem
  tuner1 : Gain
  ua_c,dc : Outport
  wires:
  tuner1/1 -> ua_c,dc/1
  Saturation3/1 -> Product/2
  Saturation1/1 -> Product2/2
  Product/1 -> pid_fb/1, Add4/1  "p"
  Product2/1 -> pid_fb/3, Add4/3  "d"
  Add4/1 -> tuner1/1, pid_fb/4  "fb"
  e_phi_dot/1 -> Saturation1/1
  Product1/1 -> Discrete-Time Integrator/1
  Discrete-Time Integrator/1 -> pid_fb/2, Add4/2  "i"
  Constant/1 -> Mux/1
  Constant1/1 -> Mux/2
  Constant2/1 -> Mux/3
  Constant4/1 -> Mux1/2
  Constant3/1 -> Mux1/1
  Constant5/1 -> Mux1/3
  pulling flag/1 -> smooth switch/3(switch)
  Mux1/1 -> smooth switch/1(u 1)
  Mux/1 -> smooth switch/2(u 2)
  smooth switch/1(y) -> Demux/1
  Demux/1 -> Product/1
  e_phi/1 -> Saturation3/1, Product1/2
  Demux/2 -> Product1/1
  Demux/3 -> Product2/1

== system ML_UAV_3D_2/UAV controller/u_r_p_Lyapunov radial position2/u_r, uav-buoy relative  position controller ==
  note: u_r feedback, uav-buoy relative position controller
  er : Inport
  integral reset : Inport  Port=2
  er_dot : Inport  Port=3
  Enable : EnablePort
  Add3 : Sum  Inputs=3
  Discrete-Time Integrator2 : DiscreteIntegrator  ExternalReset=level  SampleTime=-1  LimitOutput=on  UpperSaturationLimit=10  LowerSaturationLimit=-10  ICPrevOutput=DiscIntNeverNeededParam  ICPrevScaledInput=DiscIntNeverNeededParam
  Gain1 : Gain  Gain=controller.gains.r.ki
  Gain10 : Gain  Gain=controller.gains.r.kd
  Gain7 : Gain  Gain=controller.gains.r.kp
  Mux8 : Mux
  Saturation1 : Saturate  UpperLimit=controller.bounds.e_r_dot_max  LowerLimit=-controller.bounds.e_r_dot_max
  Saturation3 : Saturate  UpperLimit=controller.bounds.e_r_max  LowerLimit=-controller.bounds.e_r_max
  tuner : Gain
  "ur, pid_fb" : Scope
  "ur, pid_fb1" : Scope
  ur_dc : Outport
  wires:
  Discrete-Time Integrator2/1 -> Mux8/2, Add3/2
  Gain10/1 -> Mux8/3, Add3/3
  Gain1/1 -> Discrete-Time Integrator2/1
  er/1 -> Saturation3/1
  integral reset/1 -> "ur, pid_fb1"/1, Discrete-Time Integrator2/2
  Gain7/1 -> Mux8/1, Add3/1
  Add3/1 -> Mux8/4, tuner/1
  Mux8/1 -> "ur, pid_fb"/1
  tuner/1 -> ur_dc/1
  er_dot/1 -> Saturation1/1
  Saturation3/1 -> Gain1/1, Gain7/1
  Saturation1/1 -> Gain10/1

== system ML_UAV_3D_2/UAV controller/u_r_p_Lyapunov radial position3/output conditioning ==
  U_in : Inport
  switch : Inport  Port=2
  Demux : Demux  Outputs=3
  Mux3 : Mux  Inputs=3
  Subsystem1 : Subsystem
  smooth lower bound2 : Subsystem
  smooth switching with memory : Subsystem
  U_out : Outport
  wires:
  U_in/1 -> Demux/1
  switch/1 -> smooth switching with memory/2(switch), Subsystem1/1(switch)
  Demux/1 -> Subsystem1/2(u_r)  "u1"
  Demux/3 -> Mux3/3  "u3"
  smooth lower bound2/1(sat(u)) -> Mux3/2
  Demux/2 -> smooth lower bound2/1(u)  "u2"
  Subsystem1/1(Out1) -> Mux3/1
  Mux3/1 -> smooth switching with memory/1(u)
  smooth switching with memory/1(y) -> U_out/1

== system ML_UAV_3D_2/UAV controller/u_r_p_Lyapunov radial position3/u_alpha, both controllers ==
  note: Decoupled
  note: Coupled
  note: u_alpha feedback, both controllers
  e_alpha : Inport
  e_alpha_dot : Inport  Port=2
  pulling flag : Inport  Port=3
  Add4 : Sum  Inputs=3
  Constant : Constant  Value=controller.gains.alpha.kp*1.5
  Constant1 : Constant  Value=controller.gains.alpha.ki*2
  Constant2 : Constant  Value=controller.gains.alpha.kd*0.5
  Constant3 : Constant  Value=controller.gains.alpha.kp
  Constant4 : Constant  Value=controller.gains.alpha.ki
  Constant5 : Constant  Value=controller.gains.alpha.kd*1.5
  Demux : Demux  Outputs=3
  Discrete-Time Integrator : DiscreteIntegrator  SampleTime=-1  LimitOutput=on  UpperSaturationLimit=1  LowerSaturationLimit=-1  ICPrevOutput=DiscIntNeverNeededParam  ICPrevScaledInput=DiscIntNeverNeededParam
  Mux : Mux  Inputs=3
  Mux1 : Mux  Inputs=3
  Product : Product
  Product1 : Product
  Product2 : Product
  Saturation1 : Saturate  UpperLimit=7  LowerLimit=-7
  Saturation3 : Saturate  UpperLimit=7*3.14/180  LowerLimit=-7*3.14/180
  pid_fb : Scope  NumInputPorts=4
  smooth switch : Subsystem
  tuner1 : Gain
  ua_c,dc : Outport
  wires:
  tuner1/1 -> ua_c,dc/1
  Saturation3/1 -> Product/2
  Saturation1/1 -> Product2/2
  Product/1 -> pid_fb/1, Add4/1  "p"
  Product2/1 -> pid_fb/3, Add4/3  "d"
  Add4/1 -> tuner1/1, pid_fb/4  "fb"
  e_alpha_dot/1 -> Saturation1/1
  Product1/1 -> Discrete-Time Integrator/1
  Discrete-Time Integrator/1 -> pid_fb/2, Add4/2  "i"
  Constant/1 -> Mux/1
  Constant1/1 -> Mux/2
  Constant2/1 -> Mux/3
  Constant4/1 -> Mux1/2
  Constant3/1 -> Mux1/1
  Constant5/1 -> Mux1/3
  pulling flag/1 -> smooth switch/3(switch)
  Mux1/1 -> smooth switch/1(u 1)
  Mux/1 -> smooth switch/2(u 2)
  smooth switch/1(y) -> Demux/1
  Demux/1 -> Product/1
  e_alpha/1 -> Saturation3/1, Product1/2
  Demux/2 -> Product1/1
  Demux/3 -> Product2/1

== system ML_UAV_3D_2/UAV controller/u_r_p_Lyapunov radial position3/u_phi,  uav-buoy relative  position controller ==
  note: u_phi feedback, uav-buoy relative position controller
  e_phi : Inport
  integral reset : Inport  Port=2
  e_phi_dot : Inport  Port=3
  Enable : EnablePort
  Add2 : Sum  Inputs=3
  Discrete-Time Integrator3 : DiscreteIntegrator  ExternalReset=level  SampleTime=-1  LimitOutput=on  UpperSaturationLimit=1  LowerSaturationLimit=-1  ICPrevOutput=DiscIntNeverNeededParam  ICPrevScaledInput=DiscIntNeverNeededParam
  Gain12 : Gain  Gain=controller.gains.phi.ki
  Gain5 : Gain  Gain=controller.gains.phi.kd
  Gain6 : Gain  Gain=controller.gains.phi.kp
  Saturation7 : Saturate  UpperLimit=controller.bounds.e_phi_dot_dc_max  LowerLimit=-controller.bounds.e_phi_dot_dc_max
  Saturation8 : Saturate  UpperLimit=controller.bounds.e_phi_dc_max  LowerLimit=-controller.bounds.e_phi_dc_max
  pid_fb1 : Scope  NumInputPorts=4
  tuner2 : Gain
  u_phi : Outport
  wires:
  tuner2/1 -> u_phi/1
  Gain6/1 -> pid_fb1/1, Add2/1  "p"
  Gain5/1 -> Add2/3, pid_fb1/3  "d"
  Gain12/1 -> Discrete-Time Integrator3/1
  Saturation7/1 -> Gain5/1
  Add2/1 -> pid_fb1/4, tuner2/1  "fb"
  Discrete-Time Integrator3/1 -> Add2/2, pid_fb1/2  "i"
  e_phi/1 -> Saturation8/1, Gain12/1
  Saturation8/1 -> Gain6/1
  e_phi_dot/1 -> Saturation7/1
  integral reset/1 -> Discrete-Time Integrator3/2

== system ML_UAV_3D_2/UAV controller/u_r_p_Lyapunov radial position3/u_r, uav-buoy relative  position controller ==
  note: u_r feedback, uav-buoy relative position controller
  er : Inport
  integral reset : Inport  Port=2
  er_dot : Inport  Port=3
  Enable : EnablePort
  Add3 : Sum  Inputs=3
  Discrete-Time Integrator2 : DiscreteIntegrator  ExternalReset=level  SampleTime=-1  LimitOutput=on  UpperSaturationLimit=10  LowerSaturationLimit=-10  ICPrevOutput=DiscIntNeverNeededParam  ICPrevScaledInput=DiscIntNeverNeededParam
  Gain1 : Gain  Gain=controller.gains.r.ki
  Gain10 : Gain  Gain=controller.gains.r.kd
  Gain7 : Gain  Gain=controller.gains.r.kp
  Mux8 : Mux
  Saturation1 : Saturate  UpperLimit=controller.bounds.e_r_dot_max  LowerLimit=-controller.bounds.e_r_dot_max
  Saturation3 : Saturate  UpperLimit=controller.bounds.e_r_max  LowerLimit=-controller.bounds.e_r_max
  tuner : Gain
  "ur, pid_fb" : Scope
  "ur, pid_fb1" : Scope
  ur_dc : Outport
  wires:
  Discrete-Time Integrator2/1 -> Mux8/2, Add3/2
  Gain10/1 -> Mux8/3, Add3/3
  Gain1/1 -> Discrete-Time Integrator2/1
  er/1 -> Saturation3/1
  integral reset/1 -> "ur, pid_fb1"/1, Discrete-Time Integrator2/2
  Gain7/1 -> Mux8/1, Add3/1
  Add3/1 -> Mux8/4, tuner/1
  Mux8/1 -> "ur, pid_fb"/1
  tuner/1 -> ur_dc/1
  er_dot/1 -> Saturation1/1
  Saturation3/1 -> Gain1/1, Gain7/1
  Saturation1/1 -> Gain10/1

== system ML_UAV_3D_2/UAV controller/u_r_p_Lyapunov radial position3/u_x, buoy surge velocity controller ==
  note: (this is an augmentation
      | to the nominal controller
      | for better drag compensation
      | [error in tension estimation])
  note: u_x feedback, buoy surge velocity controller
  ex dot : Inport
  coupled : Inport  Port=2
  V_bar : Inport  Port=3
  integral reset : Inport  Port=4
  Enable : EnablePort
  Add1 : Sum
  Bias : Bias  Bias=0.5
  Constant1 : Constant  Value=0
  Discrete-Time Integrator1 : DiscreteIntegrator  ExternalReset=level  SampleTime=-1  LimitOutput=on  UpperSaturationLimit=10  LowerSaturationLimit=-10  ICPrevOutput=DiscIntNeverNeededParam  ICPrevScaledInput=DiscIntNeverNeededParam
  Gain11 : Gain  Gain=controller.gains.xy.ki
  Gain3 : Gain  Gain=0.5
  Gain4 : Gain  Gain=controller.gains.xy.kp
  Mux7 : Mux  Inputs=3
  Product4 : Product
  Product6 : Product
  Saturation4 : Saturate  UpperLimit=5  LowerLimit=1
  "[-22 m_u, 22 m_u]" : Saturate  UpperLimit=22.2*uav.m  LowerLimit=-22.2*uav.m
  smooth switch : Subsystem
  tuner3 : Gain
  "ur,c, PI, fb" : Scope
  "ur_c_feedback " : Scope
  ux_c : Outport
  wires:
  tuner3/1 -> "[-22 m_u, 22 m_u]"/1
  V_bar/1 -> Saturation4/1
  integral reset/1 -> smooth switch/3(switch), Discrete-Time Integrator1/2
  Add1/1 -> Mux7/3, Product4/1
  Gain3/1 -> Bias/1
  Product6/1 -> Gain11/1, Gain4/1
  Product4/1 -> tuner3/1
  Discrete-Time Integrator1/1 -> smooth switch/1(u 1)
  Bias/1 -> Product6/2
  smooth switch/1(y) -> Mux7/2, Add1/2
  ex dot/1 -> Product6/1
  "[-22 m_u, 22 m_u]"/1 -> ux_c/1, "ur_c_feedback "/1
  Saturation4/1 -> Product4/2
  Constant1/1 -> smooth switch/2(u 2)
  Gain4/1 -> Mux7/1, Add1/1
  Gain11/1 -> Discrete-Time Integrator1/1
  Mux7/1 -> "ur,c, PI, fb"/1
  coupled/1 -> Gain3/1

== system ML_UAV_3D_2/UAV controller/u_r_p_Lyapunov radial position3/u_y, buoy surge velocity controller ==
  note: u_y feedback, buoy surge velocity controller
  note: (this is an augmentation
      | to the nominal controller
      | for better drag compensation
      | [error in tension estimation])
  ey dot : Inport
  coupled : Inport  Port=2
  V_bar : Inport  Port=3
  integral reset : Inport  Port=4
  Enable : EnablePort
  Add5 : Sum
  Bias1 : Bias  Bias=0.5
  Constant2 : Constant  Value=0
  Discrete-Time Integrator4 : DiscreteIntegrator  ExternalReset=level  SampleTime=-1  LimitOutput=on  UpperSaturationLimit=10  LowerSaturationLimit=-10  ICPrevOutput=DiscIntNeverNeededParam  ICPrevScaledInput=DiscIntNeverNeededParam
  Gain13 : Gain  Gain=controller.gains.xy.ki
  Gain14 : Gain  Gain=0.5
  Gain15 : Gain  Gain=controller.gains.xy.kp
  Mux1 : Mux  Inputs=3
  Product3 : Product
  Product5 : Product
  Saturation9 : Saturate  UpperLimit=5  LowerLimit=1
  Scope1 : Scope
  "[-22 m_u, 22 m_u]1" : Saturate  UpperLimit=22.2*uav.m  LowerLimit=-22.2*uav.m
  smooth switch1 : Subsystem
  tuner4 : Gain
  "ur,c, PI, fb1" : Scope
  ur_c_feedback 1 : Scope
  uy_c : Outport
  wires:
  integral reset/1 -> smooth switch1/3(switch), Discrete-Time Integrator4/2, Scope1/1
  Discrete-Time Integrator4/1 -> smooth switch1/1(u 1)
  Saturation9/1 -> Product3/2
  Constant2/1 -> smooth switch1/2(u 2)
  Add5/1 -> Mux1/3, Product3/1
  Gain13/1 -> Discrete-Time Integrator4/1
  Product5/1 -> Gain13/1, Gain15/1
  "[-22 m_u, 22 m_u]1"/1 -> uy_c/1, ur_c_feedback 1/1
  tuner4/1 -> "[-22 m_u, 22 m_u]1"/1
  Gain15/1 -> Mux1/1, Add5/1
  smooth switch1/1(y) -> Mux1/2, Add5/2
  Mux1/1 -> "ur,c, PI, fb1"/1
  Gain14/1 -> Bias1/1
  Product3/1 -> tuner4/1
  Bias1/1 -> Product5/2
  ey dot/1 -> Product5/1
  coupled/1 -> Gain14/1
  V_bar/1 -> Saturation9/1

== system ML_UAV_3D_2/Quadrotor+buoy/6-DOF equations of motion Earth frame/D_1-5/Water Daming ==
  Rb : Inport
  Rb_T : Inport  Port=2
  eta_dot_tilde : Inport  Port=3
  dh : Inport  Port=4
  Abs : Abs
  Abs3 : Abs
  Bias : Bias  Bias=h_b/2
  Bias2 : Bias  Bias=[b_ii(1) b_ii(2) b_ii(3)]
  C_S : Fcn  Expr=0.075/(log10(u(1))-2)^2
  C_S Lewis1988 : Fcn  Expr=0.075/(log10(u(1))-2)^2
  C_S1 : Fcn  Expr=0.075/(log10(u(1))-2)^2
  Constant1 : Constant  Value=0.5*rho_w
  Constant3 : Constant  Commented=on  Value=C_S
  Create Diagonal Matrix : dspmtrx3/Create Diagonal Matrix
      settings: SourceProductName=DSP System Toolbox  SourceProductBaseCode=DS
  Gain1 : Gain  Gain=2*l_b
  Manual Switch : ManualSwitch  CurrentSetting=0
  Math Function1 : Math  Operator=transpose  SaturateOnIntegerOverflow=on
  Math Function2 : Math  Operator=transpose  SaturateOnIntegerOverflow=on
  Mux : Mux  Inputs=3
  Product1 : Product  Inputs=4
  Rb_T1 : InportShadow  Port=2
  Re Reynolds number : Gain  Gain=l_b/nu_w
  Re_Vbx : Selector  InputPortWidth=3  IndexOptions=Index vector (dialog)  Indices=1  OutputSizes=1
  Re_Vby : Selector  InputPortWidth=3  IndexOptions=Index vector (dialog)  Indices=2  OutputSizes=1
  Re_Vbz : Selector  InputPortWidth=3  IndexOptions=Index vector (dialog)  Indices=3  OutputSizes=1
  Saturation : Saturate  UpperLimit=h_b  LowerLimit=0
  Saturation1 : Saturate  UpperLimit=[inf inf inf]  LowerLimit=[0.5*10^5 0.5*10^5 0.5*10^5]
  Scope2 : Scope
  Scope5 : Scope
  Scope6 : Scope
  Selector : Selector  InputPortWidth=5  IndexOptions=Index vector (dialog)  Indices=[1 2 3]  OutputSizes=1
  Signal Specification1 : SignalSpecification  Dimensions=1
  Signal Specification2 : SignalSpecification  Dimensions=1
  Signal Specification3 : SignalSpecification  Dimensions=1
  Sum5 : Sum  Inputs=|++  SaturateOnIntegerOverflow=on
  bottom plan : Constant  Value=l_b*h_b
  buoy damping matric : Subsystem
  "tilde{nu}_12" : Product  Multiplication=Matrix(*)
  D11_I : Outport
  D12_I : Outport  Port=2
  D13_I : Outport  Port=3
  D22_I : Outport  Port=4
  D23_I : Outport  Port=5
  D33_I : Outport  Port=6
  wires:
  eta_dot_tilde/1 -> Selector/1
  Rb_T/1 -> "tilde{nu}_12"/1
  dh/1 -> Bias/1
  Gain1/1 -> Sum5/1
  bottom plan/1 -> Sum5/2
  Sum5/1 -> Product1/3  "Aw"
  Constant1/1 -> Product1/4
  Manual Switch/1 -> Product1/2  "C_S"
  "tilde{nu}_12"/1 -> Abs3/1
  Re Reynolds number/1 -> Scope6/1, Saturation1/1
  Constant3/1 -> Manual Switch/1
  C_S Lewis1988/1 -> Mux/3
  C_S/1 -> Mux/1
  Bias/1 -> Scope5/1, Saturation/1
  Saturation/1 -> Gain1/1
  Re_Vbx/1 -> C_S/1
  Re_Vbz/1 -> C_S Lewis1988/1
  Saturation1/1 -> Re_Vby/1, Re_Vbz/1, Re_Vbx/1
  Selector/1 -> "tilde{nu}_12"/2, Abs/1  "don't put the |.| here!!"
  Abs3/1 -> Product1/1  "nu_tilde_bar"
  Abs/1 -> Re Reynolds number/1
  Mux/1 -> Math Function2/1
  Re_Vby/1 -> C_S1/1
  C_S1/1 -> Mux/2
  Product1/1 -> Bias2/1
  Rb/1 -> buoy damping matric/1(Rb)
  Create Diagonal Matrix/1 -> buoy damping matric/3(D_b')
  buoy damping matric/1(D11_I) -> Signal Specification1/1
  buoy damping matric/6(D33_I) -> Signal Specification3/1
  buoy damping matric/5(D23_I) -> D23_I/1
  buoy damping matric/4(D22_I) -> Signal Specification2/1
  buoy damping matric/3(D13_I) -> D13_I/1
  buoy damping matric/2(D12_I) -> D12_I/1
  Signal Specification1/1 -> D11_I/1
  Signal Specification2/1 -> D22_I/1
  Signal Specification3/1 -> D33_I/1
  Bias2/1 -> Math Function1/1
  Math Function2/1 -> Manual Switch/2, Scope2/1
  Math Function1/1 -> Create Diagonal Matrix/1
  Rb_T1/1 -> buoy damping matric/2(Rb_T)

== system ML_UAV_3D_2/Quadrotor+buoy/6-DOF equations of motion Earth frame/D_1-5/Water Daming (simplified ==
  euler_b : Inport
  Constant1 : Constant  Value=[D_b(1) D_b(2) D_b(3)]
  Create Diagonal Matrix : dspmtrx3/Create Diagonal Matrix
      settings: SourceProductName=DSP System Toolbox  SourceProductBaseCode=DS
  buoy damping : Subsystem
  D11_I : Outport
  D12_I : Outport  Port=2
  D13_I : Outport  Port=3
  D22_I : Outport  Port=4
  D23_I : Outport  Port=5
  D33_I : Outport  Port=6
  wires:
  buoy damping/1(D11_I) -> D11_I/1
  buoy damping/4(D22_I) -> D22_I/1
  Create Diagonal Matrix/1 -> buoy damping/2(D_b')
  Constant1/1 -> Create Diagonal Matrix/1
  euler_b/1 -> buoy damping/1(euler_b)
  buoy damping/2(D12_I) -> D12_I/1
  buoy damping/3(D13_I) -> D13_I/1
  buoy damping/6(D33_I) -> D33_I/1
  buoy damping/5(D23_I) -> D23_I/1
